simulink model "n_metro_discret"  (Simulink 7.2)
settings: Solver=ode45  StartTime=0.0  StopTime=L  RelTol=1e-6
values from neighbouring files (symbols this model uses):
  Amax = Vmax/tpsm    (= 500)    [lance_crash.m]
  Delta = 10    [lance_crash.m]
  K = (randn(N,1)*sigma_K)+Knom    [lance_crash.m]
  Ka = Kry(:,dim-1:dim:dim*N)    [lance_crash.m]
  Ki = Kry(:,1:dim:dim*N)*(dim-2)    [lance_crash.m]
  Kv = Kry(:,dim:dim:dim*N)    [lance_crash.m]
  L = tdd+tpsm+2    (= 36)    [lance_crash.m]
  M_ecart = 0    [lance_crash.m]
  N = 3    [lance_crash.m]
  Tau = (randn(N,1)*sigma_Tau)+Taunom    [lance_crash.m]
  tda = 0.5    [lance_crash.m]
  tdd = Dist/Vmax    (= 32)    [lance_crash.m]
  Te = 2E-3    (= 0.002)    [lance_crash.m]
  tpsm = 2    [lance_crash.m]
undefined symbols (not defined in the file or in its folder): DiscIntNeverNeededParam
settings Model: Creator=acco  LastModifiedBy=acco
settings DataIOCC: SignalLoggingName=sigsOut
settings DebuggingCC: SaveWithParameterizedLinksMsg=none  SignalResolutionControl=TryResolveAllWithWarning  SolverPrmCheckMsg=none  MultiTaskDSMMsg=warning  MultiTaskCondExecSysMsg=none  StrictBusMsg=None
settings HardwareCC: TargetUnknown=on
settings RTWCC: IncludeERTFirstTime=on

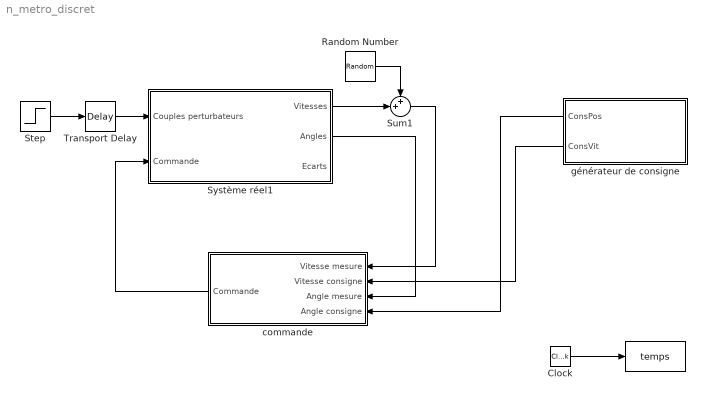
== system n_metro_discret ==
  " " : ToWorkspace  VariableName=temps  SampleTime=Te  SaveFormat=Array
  Clock : DigitalClock  SampleTime=Te
  Random Number : RandomNumber  Mean=zeros(N,1)  Variance=ones(N,1)*50  Seed=rand(N,1)  SampleTime=Te
  Step : Step  Time=L*0.1  Before=ones(N,1)*0  After=-ones(N,1)*0
  Sum1 : Sum  Inputs=++|  OutDataType=sfix(16)  OutScaling=2^0  SaturateOnIntegerOverflow=on
  Système réel1 : Subsystem
  Transport Delay : TransportDelay  DelayTime=N-(1:N)
  commande : Subsystem  Orientation=left  TreatAsAtomicUnit=on
      settings: RTWSystemCode=Function  RTWFcnNameOpts=Use subsystem name  RTWFileNameOpts=Use subsystem name
  générateur de consigne : Subsystem  Orientation=left
  wires:
  Step/1 -> Transport Delay/1
  Système réel1/2(Angles) -> commande/3(Angle mesure)
  Clock/1 -> " "/1
  commande/1(Commande) -> Système réel1/2(Commande)
  générateur de consigne/1(ConsPos) -> commande/4(Angle consigne)
  Transport Delay/1 -> Système réel1/1(Couples perturbateurs)
  générateur de consigne/2(ConsVit) -> commande/2(Vitesse consigne)
  Système réel1/1(Vitesses) -> Sum1/2
  Sum1/1 -> commande/1(Vitesse mesure)
  Random Number/1 -> Sum1/1

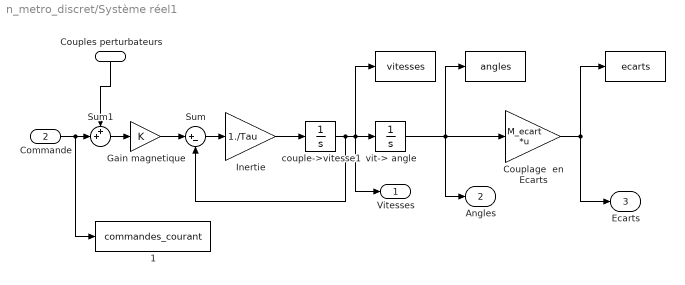
== system n_metro_discret/Système réel1 ==
  Couples perturbateurs : Inport  Orientation=down  OutDataType=sfix(16)  OutScaling=2^0
  Commande : Inport  Port=2  OutDataType=sfix(16)  OutScaling=2^0
  " " : ToWorkspace  VariableName=vitesses  SampleTime=Te  SaveFormat=Array
  "  " : ToWorkspace  VariableName=angles  SampleTime=Te  SaveFormat=Array
  "   " : ToWorkspace  VariableName=ecarts  SampleTime=Te  SaveFormat=Array
  "   1" : ToWorkspace  VariableName=commandes_courant  SampleTime=Te  SaveFormat=Array
  Couplage  en Ecarts : Gain  Gain=M_ecart  Multiplication=Matrix(K*u)  ParameterDataType=sfix(16)  ParameterScaling=2^0  OutDataType=sfix(16)  OutScaling=2^0  SaturateOnIntegerOverflow=on  OutDataTypeStr=Inherit: Same as input  ParamDataTypeStr=Inherit: Same as input
  Gain magnetique : Gain  Gain=K  ParameterDataType=sfix(16)  ParameterScaling=2^0  OutDataType=sfix(16)  OutScaling=2^0  SaturateOnIntegerOverflow=on  OutDataTypeStr=Inherit: Same as input  ParamDataTypeStr=Inherit: Same as input
  Inertie : Gain  Gain=1./Tau  ParameterDataType=sfix(16)  ParameterScaling=2^0  OutDataType=sfix(16)  OutScaling=2^0  SaturateOnIntegerOverflow=on  OutDataTypeStr=Inherit: Same as input  ParamDataTypeStr=Inherit: Same as input
  Sum : Sum  Inputs=|+-  OutDataType=sfix(16)  OutScaling=2^0  SaturateOnIntegerOverflow=on
  Sum1 : Sum  Inputs=++|  OutDataType=sfix(16)  OutScaling=2^0  SaturateOnIntegerOverflow=on
  couple->vitesse1 : Integrator  InitialCondition=zeros(N,1)
  vit-> angle : Integrator  InitialCondition=(0:N-1)*Delta
  Vitesses : Outport  OutDataType=sfix(16)  OutScaling=2^0
  Angles : Outport  Port=2  OutDataType=sfix(16)  OutScaling=2^0
  Ecarts : Outport  Port=3  OutDataType=sfix(16)  OutScaling=2^0
  wires:
  vit-> angle/1 -> "  "/1, Angles/1, Couplage  en Ecarts/1
  Commande/1 -> "   1"/1, Sum1/2
  Couplage  en Ecarts/1 -> "   "/1, Ecarts/1
  Inertie/1 -> couple->vitesse1/1
  Gain magnetique/1 -> Sum/1
  Sum/1 -> Inertie/1
  couple->vitesse1/1 -> vit-> angle/1, Vitesses/1, " "/1, Sum/2
  Sum1/1 -> Gain magnetique/1
  Couples perturbateurs/1 -> Sum1/1

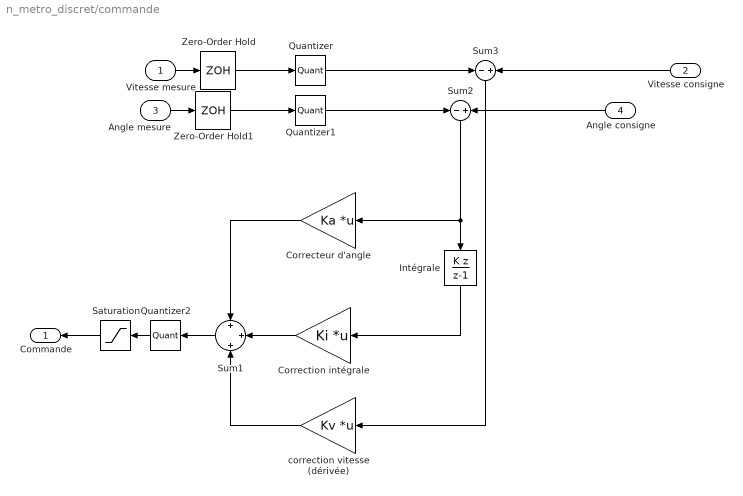
== system n_metro_discret/commande ==
  Vitesse mesure : Inport  OutDataType=sfix(16)  OutScaling=2^0
  Vitesse consigne : Inport  Orientation=left  Port=2  OutDataType=sfix(16)  OutScaling=2^0
  Angle mesure : Inport  Port=3  OutDataType=sfix(16)  OutScaling=2^0
  Angle consigne : Inport  Orientation=left  Port=4  OutDataType=sfix(16)  OutScaling=2^0
  Correcteur d'angle : Gain  Orientation=left  Gain=Ka  Multiplication=Matrix(K*u)  ParameterDataType=sfix(16)  ParameterScaling=2^0  OutDataType=sfix(16)  OutScaling=2^0  SaturateOnIntegerOverflow=on  OutDataTypeStr=Inherit: Same as input  ParamDataTypeStr=Inherit: Same as input
  Correction intégrale : Gain  Orientation=left  Gain=Ki  Multiplication=Matrix(K*u)  ParameterDataType=sfix(16)  ParameterScaling=2^0  OutDataType=sfix(16)  OutScaling=2^0  SaturateOnIntegerOverflow=on  OutDataTypeStr=Inherit: Same as input  ParamDataTypeStr=Inherit: Same as input
  Intégrale : DiscreteIntegrator  Orientation=down  IntegratorMethod=Accumulation: Backward Euler  gainval=1.0*ones(N,1)  InitialCondition=zeros(N,1)  SampleTime=Te  LimitOutput=on  UpperSaturationLimit=4095/max(max(Ki))*ones(N,1)  LowerSaturationLimit=-4095/max(max(Ki))*ones(N,1)  ICPrevOutput=DiscIntNeverNeededParam  ICPrevScaledInput=DiscIntNeverNeededParam
  Quantizer : Quantizer  QuantizationInterval=1
  Quantizer1 : Quantizer  QuantizationInterval=1
  Quantizer2 : Quantizer  Orientation=left  QuantizationInterval=1
  Saturation : Saturate  Orientation=left  UpperLimit=4095  LowerLimit=-4095  OutDataType=sfix(16)  OutScaling=2^0
  Sum1 : Sum  Orientation=left  Inputs=+|+|+  OutDataType=sfix(16)  OutScaling=2^0  SaturateOnIntegerOverflow=on
  Sum2 : Sum  Orientation=down  Inputs=-|+  OutDataType=sfix(16)  OutScaling=2^0  SaturateOnIntegerOverflow=on
  Sum3 : Sum  Orientation=down  Inputs=-|+  OutDataType=sfix(16)  OutScaling=2^0  SaturateOnIntegerOverflow=on
  Zero-Order Hold : ZeroOrderHold  SampleTime=Te
  Zero-Order Hold1 : ZeroOrderHold  SampleTime=Te
  correction vitesse (dérivée) : Gain  Orientation=left  Gain=Kv  Multiplication=Matrix(K*u)  ParameterDataType=sfix(16)  ParameterScaling=2^0  OutDataType=sfix(16)  OutScaling=2^0  SaturateOnIntegerOverflow=on  OutDataTypeStr=Inherit: Same as input  ParamDataTypeStr=Inherit: Same as input
  Commande : Outport  Orientation=left
  wires:
  Sum2/1 -> Intégrale/1, Correcteur d'angle/1
  Correcteur d'angle/1 -> Sum1/1
  Sum3/1 -> correction vitesse (dérivée)/1
  Intégrale/1 -> Correction intégrale/1
  correction vitesse (dérivée)/1 -> Sum1/3
  Correction intégrale/1 -> Sum1/2
  Vitesse consigne/1 -> Sum3/2
  Angle consigne/1 -> Sum2/2
  Vitesse mesure/1 -> Zero-Order Hold/1
  Angle mesure/1 -> Zero-Order Hold1/1
  Sum1/1 -> Quantizer2/1
  Zero-Order Hold/1 -> Quantizer/1
  Zero-Order Hold1/1 -> Quantizer1/1
  Saturation/1 -> Commande/1
  Quantizer/1 -> Sum3/1
  Quantizer1/1 -> Sum2/1
  Quantizer2/1 -> Saturation/1

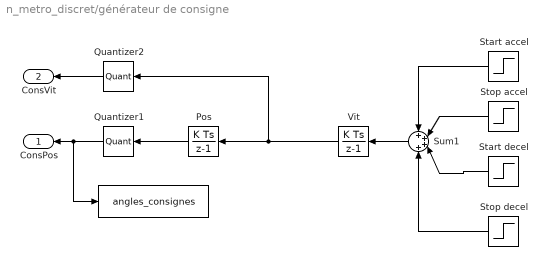
== system n_metro_discret/générateur de consigne ==
  "  " : ToWorkspace  VariableName=angles_consignes  SampleTime=Te  SaveFormat=Array
  Pos : DiscreteIntegrator  Orientation=left  InitialCondition=[0:N-1]'*Delta  SampleTime=Te  ICPrevOutput=DiscIntNeverNeededParam  ICPrevScaledInput=DiscIntNeverNeededParam
  Quantizer1 : Quantizer  Orientation=left  QuantizationInterval=1
  Quantizer2 : Quantizer  Orientation=left  QuantizationInterval=1
  Start accel : Step  Orientation=left  Time=tda  Before=ones(N,1)*0  After=ones(N,1)*Amax  SampleTime=Te
  Start decel : Step  Orientation=left  Time=tdd  Before=ones(N,1)*0  After=-ones(N,1)*Amax  SampleTime=Te
  Stop accel : Step  Orientation=left  Time=tda+tpsm  Before=ones(N,1)*0  After=-ones(N,1)*Amax  SampleTime=Te
  Stop decel : Step  Orientation=left  Time=tdd+tpsm  Before=ones(N,1)*0  After=ones(N,1)*Amax  SampleTime=Te
  Sum1 : Sum  Orientation=left  Inputs=++++  OutDataType=sfix(16)  OutScaling=2^0  SaturateOnIntegerOverflow=on
  Vit : DiscreteIntegrator  Orientation=left  InitialCondition=ones(N,1)*0  SampleTime=Te  ICPrevOutput=DiscIntNeverNeededParam  ICPrevScaledInput=DiscIntNeverNeededParam
  ConsPos : Outport  Orientation=left
  ConsVit : Outport  Orientation=left  Port=2
  wires:
  Vit/1 -> Pos/1, Quantizer2/1
  Pos/1 -> Quantizer1/1
  Start accel/1 -> Sum1/1
  Stop accel/1 -> Sum1/2
  Start decel/1 -> Sum1/3
  Stop decel/1 -> Sum1/4
  Sum1/1 -> Vit/1
  Quantizer2/1 -> ConsVit/1
  Quantizer1/1 -> "  "/1, ConsPos/1
